simulink model "tracker"  (R2020a)
settings: Solver=VariableStepAuto  StartTime=0.0  StopTime=simulation_time  RelTol=1e-3
values from neighbouring files (symbols this model uses):
  costas_pll_arctan_nstage = 8    [tracker_hw_init.m]
  costas_pll_arctan_point = 16    [tracker_hw_init.m]
  costas_pll_arctan_width = 32    [tracker_hw_init.m]
  DDS_ch_pinc = fc.*(2^(DDS_phase_width)/fs)    [tracker_hw_init.m]
  fs = 120e6    (= 120000000)    [tracker_hw_init.m]
  normalized_EML_power_cordic_nstage = 11    [tracker_hw_init.m]
  normalized_EML_power_cordic_point = 32    [tracker_hw_init.m]
  normalized_EML_power_cordic_width = 32    [tracker_hw_init.m]
  ts = 1/fs    (= 8.33333333333e-09)    [tracker_hw_init.m]
undefined symbols (not defined in the file or in its folder): cacode, i
libraries: xbsIndex_r4 x1873
(part 2 of 14)

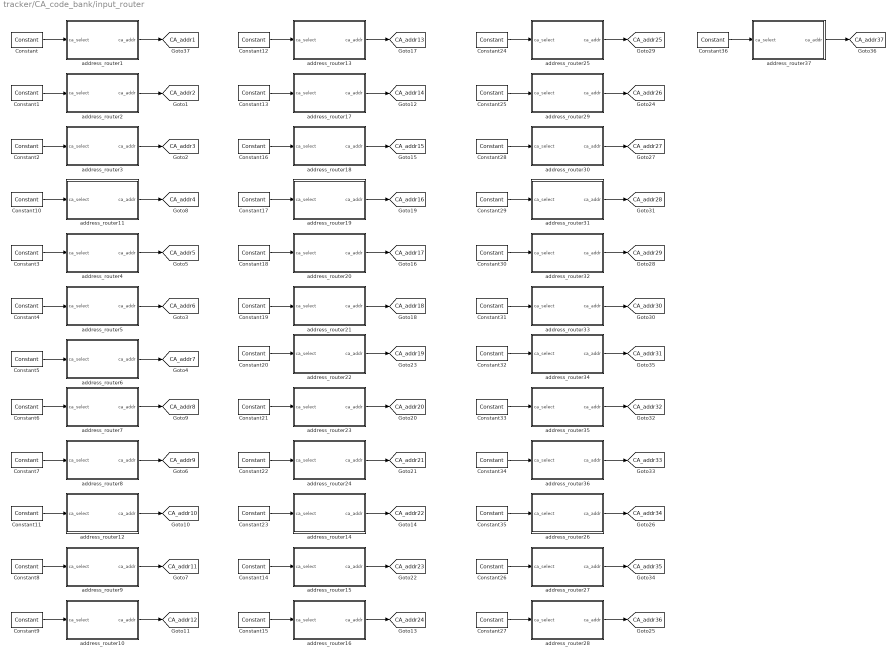
== system tracker/CA_code_bank/input_router ==
  Constant : xbsIndex_r4/Constant  const=0  gui_display_data_type=Fixed-point  arith_type=Unsigned  n_bits=6  bin_pt=0  preci_type=Single  exp_width=8  frac_width=24  explicit_period=off  period=1  equ=P=C  opselect=C  inp2=PCIN>>17  opr=+  inp1=P  carry=CIN  dbl_ovrd=off  block_type=constant
  Constant1 : xbsIndex_r4/Constant  const=1.0  gui_display_data_type=Fixed-point  arith_type=Unsigned  n_bits=6  bin_pt=0  preci_type=Single  exp_width=8  frac_width=24  explicit_period=off  period=1  equ=P=C  opselect=C  inp2=PCIN>>17  opr=+  inp1=P  carry=CIN  dbl_ovrd=off  block_type=constant
  Constant10 : xbsIndex_r4/Constant  const=3  gui_display_data_type=Fixed-point  arith_type=Unsigned  n_bits=6  bin_pt=0  preci_type=Single  exp_width=8  frac_width=24  explicit_period=off  period=1  equ=P=C  opselect=C  inp2=PCIN>>17  opr=+  inp1=P  carry=CIN  dbl_ovrd=off  block_type=constant
  Constant11 : xbsIndex_r4/Constant  const=9  gui_display_data_type=Fixed-point  arith_type=Unsigned  n_bits=6  bin_pt=0  preci_type=Single  exp_width=8  frac_width=24  explicit_period=off  period=1  equ=P=C  opselect=C  inp2=PCIN>>17  opr=+  inp1=P  carry=CIN  dbl_ovrd=off  block_type=constant
  Constant12 : xbsIndex_r4/Constant  const=12  gui_display_data_type=Fixed-point  arith_type=Unsigned  n_bits=6  bin_pt=0  preci_type=Single  exp_width=8  frac_width=24  explicit_period=off  period=1  equ=P=C  opselect=C  inp2=PCIN>>17  opr=+  inp1=P  carry=CIN  dbl_ovrd=off  block_type=constant
  Constant13 : xbsIndex_r4/Constant  const=13  gui_display_data_type=Fixed-point  arith_type=Unsigned  n_bits=6  bin_pt=0  preci_type=Single  exp_width=8  frac_width=24  explicit_period=off  period=1  equ=P=C  opselect=C  inp2=PCIN>>17  opr=+  inp1=P  carry=CIN  dbl_ovrd=off  block_type=constant
  Constant14 : xbsIndex_r4/Constant  const=22  gui_display_data_type=Fixed-point  arith_type=Unsigned  n_bits=6  bin_pt=0  preci_type=Single  exp_width=8  frac_width=24  explicit_period=off  period=1  equ=P=C  opselect=C  inp2=PCIN>>17  opr=+  inp1=P  carry=CIN  dbl_ovrd=off  block_type=constant
  Constant15 : xbsIndex_r4/Constant  const=23  gui_display_data_type=Fixed-point  arith_type=Unsigned  n_bits=6  bin_pt=0  preci_type=Single  exp_width=8  frac_width=24  explicit_period=off  period=1  equ=P=C  opselect=C  inp2=PCIN>>17  opr=+  inp1=P  carry=CIN  dbl_ovrd=off  block_type=constant
  Constant16 : xbsIndex_r4/Constant  const=14  gui_display_data_type=Fixed-point  arith_type=Unsigned  n_bits=6  bin_pt=0  preci_type=Single  exp_width=8  frac_width=24  explicit_period=off  period=1  equ=P=C  opselect=C  inp2=PCIN>>17  opr=+  inp1=P  carry=CIN  dbl_ovrd=off  block_type=constant
  Constant17 : xbsIndex_r4/Constant  const=15  gui_display_data_type=Fixed-point  arith_type=Unsigned  n_bits=6  bin_pt=0  preci_type=Single  exp_width=8  frac_width=24  explicit_period=off  period=1  equ=P=C  opselect=C  inp2=PCIN>>17  opr=+  inp1=P  carry=CIN  dbl_ovrd=off  block_type=constant
  Constant18 : xbsIndex_r4/Constant  const=16  gui_display_data_type=Fixed-point  arith_type=Unsigned  n_bits=6  bin_pt=0  preci_type=Single  exp_width=8  frac_width=24  explicit_period=off  period=1  equ=P=C  opselect=C  inp2=PCIN>>17  opr=+  inp1=P  carry=CIN  dbl_ovrd=off  block_type=constant
  Constant19 : xbsIndex_r4/Constant  const=17  gui_display_data_type=Fixed-point  arith_type=Unsigned  n_bits=6  bin_pt=0  preci_type=Single  exp_width=8  frac_width=24  explicit_period=off  period=1  equ=P=C  opselect=C  inp2=PCIN>>17  opr=+  inp1=P  carry=CIN  dbl_ovrd=off  block_type=constant
  Constant2 : xbsIndex_r4/Constant  const=2  gui_display_data_type=Fixed-point  arith_type=Unsigned  n_bits=6  bin_pt=0  preci_type=Single  exp_width=8  frac_width=24  explicit_period=off  period=1  equ=P=C  opselect=C  inp2=PCIN>>17  opr=+  inp1=P  carry=CIN  dbl_ovrd=off  block_type=constant
  Constant20 : xbsIndex_r4/Constant  const=18  gui_display_data_type=Fixed-point  arith_type=Unsigned  n_bits=6  bin_pt=0  preci_type=Single  exp_width=8  frac_width=24  explicit_period=off  period=1  equ=P=C  opselect=C  inp2=PCIN>>17  opr=+  inp1=P  carry=CIN  dbl_ovrd=off  block_type=constant
  Constant21 : xbsIndex_r4/Constant  const=19  gui_display_data_type=Fixed-point  arith_type=Unsigned  n_bits=6  bin_pt=0  preci_type=Single  exp_width=8  frac_width=24  explicit_period=off  period=1  equ=P=C  opselect=C  inp2=PCIN>>17  opr=+  inp1=P  carry=CIN  dbl_ovrd=off  block_type=constant
  Constant22 : xbsIndex_r4/Constant  const=20  gui_display_data_type=Fixed-point  arith_type=Unsigned  n_bits=6  bin_pt=0  preci_type=Single  exp_width=8  frac_width=24  explicit_period=off  period=1  equ=P=C  opselect=C  inp2=PCIN>>17  opr=+  inp1=P  carry=CIN  dbl_ovrd=off  block_type=constant
  Constant23 : xbsIndex_r4/Constant  const=21  gui_display_data_type=Fixed-point  arith_type=Unsigned  n_bits=6  bin_pt=0  preci_type=Single  exp_width=8  frac_width=24  explicit_period=off  period=1  equ=P=C  opselect=C  inp2=PCIN>>17  opr=+  inp1=P  carry=CIN  dbl_ovrd=off  block_type=constant
  Constant24 : xbsIndex_r4/Constant  const=24  gui_display_data_type=Fixed-point  arith_type=Unsigned  n_bits=6  bin_pt=0  preci_type=Single  exp_width=8  frac_width=24  explicit_period=off  period=1  equ=P=C  opselect=C  inp2=PCIN>>17  opr=+  inp1=P  carry=CIN  dbl_ovrd=off  block_type=constant
  Constant25 : xbsIndex_r4/Constant  const=25  gui_display_data_type=Fixed-point  arith_type=Unsigned  n_bits=6  bin_pt=0  preci_type=Single  exp_width=8  frac_width=24  explicit_period=off  period=1  equ=P=C  opselect=C  inp2=PCIN>>17  opr=+  inp1=P  carry=CIN  dbl_ovrd=off  block_type=constant
  Constant26 : xbsIndex_r4/Constant  const=34  gui_display_data_type=Fixed-point  arith_type=Unsigned  n_bits=6  bin_pt=0  preci_type=Single  exp_width=8  frac_width=24  explicit_period=off  period=1  equ=P=C  opselect=C  inp2=PCIN>>17  opr=+  inp1=P  carry=CIN  dbl_ovrd=off  block_type=constant
  Constant27 : xbsIndex_r4/Constant  const=35  gui_display_data_type=Fixed-point  arith_type=Unsigned  n_bits=6  bin_pt=0  preci_type=Single  exp_width=8  frac_width=24  explicit_period=off  period=1  equ=P=C  opselect=C  inp2=PCIN>>17  opr=+  inp1=P  carry=CIN  dbl_ovrd=off  block_type=constant
  Constant28 : xbsIndex_r4/Constant  const=26  gui_display_data_type=Fixed-point  arith_type=Unsigned  n_bits=6  bin_pt=0  preci_type=Single  exp_width=8  frac_width=24  explicit_period=off  period=1  equ=P=C  opselect=C  inp2=PCIN>>17  opr=+  inp1=P  carry=CIN  dbl_ovrd=off  block_type=constant
  Constant29 : xbsIndex_r4/Constant  const=27  gui_display_data_type=Fixed-point  arith_type=Unsigned  n_bits=6  bin_pt=0  preci_type=Single  exp_width=8  frac_width=24  explicit_period=off  period=1  equ=P=C  opselect=C  inp2=PCIN>>17  opr=+  inp1=P  carry=CIN  dbl_ovrd=off  block_type=constant
  Constant3 : xbsIndex_r4/Constant  const=4  gui_display_data_type=Fixed-point  arith_type=Unsigned  n_bits=6  bin_pt=0  preci_type=Single  exp_width=8  frac_width=24  explicit_period=off  period=1  equ=P=C  opselect=C  inp2=PCIN>>17  opr=+  inp1=P  carry=CIN  dbl_ovrd=off  block_type=constant
  Constant30 : xbsIndex_r4/Constant  const=28  gui_display_data_type=Fixed-point  arith_type=Unsigned  n_bits=6  bin_pt=0  preci_type=Single  exp_width=8  frac_width=24  explicit_period=off  period=1  equ=P=C  opselect=C  inp2=PCIN>>17  opr=+  inp1=P  carry=CIN  dbl_ovrd=off  block_type=constant
  Constant31 : xbsIndex_r4/Constant  const=29  gui_display_data_type=Fixed-point  arith_type=Unsigned  n_bits=6  bin_pt=0  preci_type=Single  exp_width=8  frac_width=24  explicit_period=off  period=1  equ=P=C  opselect=C  inp2=PCIN>>17  opr=+  inp1=P  carry=CIN  dbl_ovrd=off  block_type=constant
  Constant32 : xbsIndex_r4/Constant  const=30  gui_display_data_type=Fixed-point  arith_type=Unsigned  n_bits=6  bin_pt=0  preci_type=Single  exp_width=8  frac_width=24  explicit_period=off  period=1  equ=P=C  opselect=C  inp2=PCIN>>17  opr=+  inp1=P  carry=CIN  dbl_ovrd=off  block_type=constant
  Constant33 : xbsIndex_r4/Constant  const=31  gui_display_data_type=Fixed-point  arith_type=Unsigned  n_bits=6  bin_pt=0  preci_type=Single  exp_width=8  frac_width=24  explicit_period=off  period=1  equ=P=C  opselect=C  inp2=PCIN>>17  opr=+  inp1=P  carry=CIN  dbl_ovrd=off  block_type=constant
  Constant34 : xbsIndex_r4/Constant  const=32  gui_display_data_type=Fixed-point  arith_type=Unsigned  n_bits=6  bin_pt=0  preci_type=Single  exp_width=8  frac_width=24  explicit_period=off  period=1  equ=P=C  opselect=C  inp2=PCIN>>17  opr=+  inp1=P  carry=CIN  dbl_ovrd=off  block_type=constant
  Constant35 : xbsIndex_r4/Constant  const=33  gui_display_data_type=Fixed-point  arith_type=Unsigned  n_bits=6  bin_pt=0  preci_type=Single  exp_width=8  frac_width=24  explicit_period=off  period=1  equ=P=C  opselect=C  inp2=PCIN>>17  opr=+  inp1=P  carry=CIN  dbl_ovrd=off  block_type=constant
  Constant36 : xbsIndex_r4/Constant  const=36  gui_display_data_type=Fixed-point  arith_type=Unsigned  n_bits=6  bin_pt=0  preci_type=Single  exp_width=8  frac_width=24  explicit_period=off  period=1  equ=P=C  opselect=C  inp2=PCIN>>17  opr=+  inp1=P  carry=CIN  dbl_ovrd=off  block_type=constant
  Constant4 : xbsIndex_r4/Constant  const=5  gui_display_data_type=Fixed-point  arith_type=Unsigned  n_bits=6  bin_pt=0  preci_type=Single  exp_width=8  frac_width=24  explicit_period=off  period=1  equ=P=C  opselect=C  inp2=PCIN>>17  opr=+  inp1=P  carry=CIN  dbl_ovrd=off  block_type=constant
  Constant5 : xbsIndex_r4/Constant  const=6  gui_display_data_type=Fixed-point  arith_type=Unsigned  n_bits=6  bin_pt=0  preci_type=Single  exp_width=8  frac_width=24  explicit_period=off  period=1  equ=P=C  opselect=C  inp2=PCIN>>17  opr=+  inp1=P  carry=CIN  dbl_ovrd=off  block_type=constant
  Constant6 : xbsIndex_r4/Constant  const=7  gui_display_data_type=Fixed-point  arith_type=Unsigned  n_bits=6  bin_pt=0  preci_type=Single  exp_width=8  frac_width=24  explicit_period=off  period=1  equ=P=C  opselect=C  inp2=PCIN>>17  opr=+  inp1=P  carry=CIN  dbl_ovrd=off  block_type=constant
  Constant7 : xbsIndex_r4/Constant  const=8  gui_display_data_type=Fixed-point  arith_type=Unsigned  n_bits=6  bin_pt=0  preci_type=Single  exp_width=8  frac_width=24  explicit_period=off  period=1  equ=P=C  opselect=C  inp2=PCIN>>17  opr=+  inp1=P  carry=CIN  dbl_ovrd=off  block_type=constant
  Constant8 : xbsIndex_r4/Constant  const=10  gui_display_data_type=Fixed-point  arith_type=Unsigned  n_bits=6  bin_pt=0  preci_type=Single  exp_width=8  frac_width=24  explicit_period=off  period=1  equ=P=C  opselect=C  inp2=PCIN>>17  opr=+  inp1=P  carry=CIN  dbl_ovrd=off  block_type=constant
  Constant9 : xbsIndex_r4/Constant  const=11  gui_display_data_type=Fixed-point  arith_type=Unsigned  n_bits=6  bin_pt=0  preci_type=Single  exp_width=8  frac_width=24  explicit_period=off  period=1  equ=P=C  opselect=C  inp2=PCIN>>17  opr=+  inp1=P  carry=CIN  dbl_ovrd=off  block_type=constant
  address_router1 : Subsystem
  address_router10 : Subsystem
  address_router11 : Subsystem
  address_router12 : Subsystem
  address_router13 : Subsystem
  address_router14 : Subsystem
  address_router15 : Subsystem
  address_router16 : Subsystem
  address_router17 : Subsystem
  address_router18 : Subsystem
  address_router19 : Subsystem
  address_router2 : Subsystem
  address_router20 : Subsystem
  address_router21 : Subsystem
  address_router22 : Subsystem
  address_router23 : Subsystem
  address_router24 : Subsystem
  address_router25 : Subsystem
  address_router26 : Subsystem
  address_router27 : Subsystem
  address_router28 : Subsystem
  address_router29 : Subsystem
  address_router3 : Subsystem
  address_router30 : Subsystem
  address_router31 : Subsystem
  address_router32 : Subsystem
  address_router33 : Subsystem
  address_router34 : Subsystem
  address_router35 : Subsystem
  address_router36 : Subsystem
  address_router37 : Subsystem
  address_router4 : Subsystem
  address_router5 : Subsystem
  address_router6 : Subsystem
  address_router7 : Subsystem
  address_router8 : Subsystem
  address_router9 : Subsystem
  tag scope: CA_addr10=global, CA_addr11=global, CA_addr12=global, CA_addr13=global, CA_addr14=global, CA_addr15=global, CA_addr16=global, CA_addr17=global, CA_addr18=global, CA_addr19=global, CA_addr1=global, CA_addr20=global, CA_addr21=global, CA_addr22=global, CA_addr23=global, CA_addr24=global, CA_addr25=global, CA_addr26=global, CA_addr27=global, CA_addr28=global, CA_addr29=global, CA_addr2=global, CA_addr30=global, CA_addr31=global, CA_addr32=global, CA_addr33=global, CA_addr34=global, CA_addr35=global, CA_addr36=global, CA_addr37=global, CA_addr3=global, CA_addr4=global, CA_addr5=global, CA_addr6=global, CA_addr7=global, CA_addr8=global, CA_addr9=global
  wires:
  address_router1/1(ca_addr) -> [CA_addr1]
  Constant/1 -> address_router1/1(ca_select)
  address_router2/1(ca_addr) -> [CA_addr2]
  Constant1/1 -> address_router2/1(ca_select)
  Constant2/1 -> address_router3/1(ca_select)
  address_router3/1(ca_addr) -> [CA_addr3]
  address_router6/1(ca_addr) -> [CA_addr7]
  Constant5/1 -> address_router6/1(ca_select)
  Constant4/1 -> address_router5/1(ca_select)
  address_router5/1(ca_addr) -> [CA_addr6]
  Constant3/1 -> address_router4/1(ca_select)
  address_router4/1(ca_addr) -> [CA_addr5]
  address_router10/1(ca_addr) -> [CA_addr12]
  Constant9/1 -> address_router10/1(ca_select)
  address_router11/1(ca_addr) -> [CA_addr4]
  Constant10/1 -> address_router11/1(ca_select)
  Constant11/1 -> address_router12/1(ca_select)
  address_router12/1(ca_addr) -> [CA_addr10]
  address_router9/1(ca_addr) -> [CA_addr11]
  Constant8/1 -> address_router9/1(ca_select)
  Constant7/1 -> address_router8/1(ca_select)
  address_router8/1(ca_addr) -> [CA_addr9]
  Constant6/1 -> address_router7/1(ca_select)
  address_router7/1(ca_addr) -> [CA_addr8]
  address_router22/1(ca_addr) -> [CA_addr19]
  Constant20/1 -> address_router22/1(ca_select)
  address_router23/1(ca_addr) -> [CA_addr20]
  Constant21/1 -> address_router23/1(ca_select)
  Constant22/1 -> address_router24/1(ca_select)
  address_router24/1(ca_addr) -> [CA_addr21]
  address_router16/1(ca_addr) -> [CA_addr24]
  Constant15/1 -> address_router16/1(ca_select)
  Constant14/1 -> address_router15/1(ca_select)
  address_router15/1(ca_addr) -> [CA_addr23]
  Constant23/1 -> address_router14/1(ca_select)
  address_router14/1(ca_addr) -> [CA_addr22]
  address_router19/1(ca_addr) -> [CA_addr16]
  Constant17/1 -> address_router19/1(ca_select)
  address_router20/1(ca_addr) -> [CA_addr17]
  Constant18/1 -> address_router20/1(ca_select)
  Constant19/1 -> address_router21/1(ca_select)
  address_router21/1(ca_addr) -> [CA_addr18]
  address_router18/1(ca_addr) -> [CA_addr15]
  Constant16/1 -> address_router18/1(ca_select)
  Constant13/1 -> address_router17/1(ca_select)
  address_router17/1(ca_addr) -> [CA_addr14]
  Constant12/1 -> address_router13/1(ca_select)
  address_router13/1(ca_addr) -> [CA_addr13]
  address_router25/1(ca_addr) -> [CA_addr25]
  Constant24/1 -> address_router25/1(ca_select)
  address_router29/1(ca_addr) -> [CA_addr26]
  Constant25/1 -> address_router29/1(ca_select)
  Constant28/1 -> address_router30/1(ca_select)
  address_router30/1(ca_addr) -> [CA_addr27]
  address_router33/1(ca_addr) -> [CA_addr30]
  Constant31/1 -> address_router33/1(ca_select)
  Constant30/1 -> address_router32/1(ca_select)
  address_router32/1(ca_addr) -> [CA_addr29]
  Constant29/1 -> address_router31/1(ca_select)
  address_router31/1(ca_addr) -> [CA_addr28]
  address_router26/1(ca_addr) -> [CA_addr34]
  Constant35/1 -> address_router26/1(ca_select)
  address_router27/1(ca_addr) -> [CA_addr35]
  Constant26/1 -> address_router27/1(ca_select)
  Constant27/1 -> address_router28/1(ca_select)
  address_router28/1(ca_addr) -> [CA_addr36]
  address_router36/1(ca_addr) -> [CA_addr33]
  Constant34/1 -> address_router36/1(ca_select)
  Constant33/1 -> address_router35/1(ca_select)
  address_router35/1(ca_addr) -> [CA_addr32]
  Constant32/1 -> address_router34/1(ca_select)
  address_router34/1(ca_addr) -> [CA_addr31]
  Constant36/1 -> address_router37/1(ca_select)
  address_router37/1(ca_addr) -> [CA_addr37]

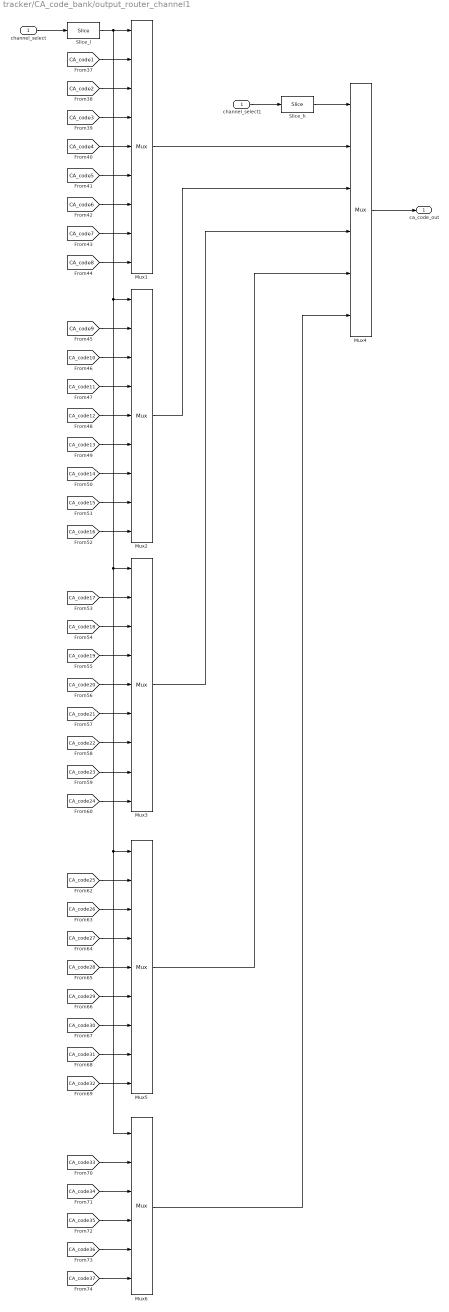
== system tracker/CA_code_bank/output_router_channel1 ==
  channel_select : Inport
  Mux{1..3,5} (4 alike) : xbsIndex_r4/Mux  inputs=8  en=off  latency=1  precision=Full  arith_type=Unsigned  n_bits=16  bin_pt=14  quantization=Truncate  overflow=Wrap  dbl_ovrd=off  block_type=mux
  Mux4 : xbsIndex_r4/Mux  inputs=5  en=off  latency=1  precision=Full  arith_type=Unsigned  n_bits=16  bin_pt=14  quantization=Truncate  overflow=Wrap  dbl_ovrd=off  block_type=mux
  Mux6 : xbsIndex_r4/Mux  inputs=5  en=off  latency=1  precision=Full  arith_type=Unsigned  n_bits=16  bin_pt=14  quantization=Truncate  overflow=Wrap  dbl_ovrd=off  block_type=mux
  Slice_h : xbsIndex_r4/Slice  nbits=3  boolean_output=off  mode=Lower Bit Location + Width  bit1=0  base1=MSB of Input  bit0=3  base0=LSB of Input  dbl_ovrd=off  block_type=slice
  Slice_l : xbsIndex_r4/Slice  nbits=3  boolean_output=off  mode=Lower Bit Location + Width  bit1=0  base1=MSB of Input  bit0=0  base0=LSB of Input  dbl_ovrd=off  block_type=slice
  channel_select1 : InportShadow
  ca_code_out : Outport
  wires:
  [CA_code10] -> Mux2/3
  [CA_code1] -> Mux1/2
  [CA_code18] -> Mux3/3
  [CA_code11] -> Mux2/4
  Mux6/1 -> Mux4/6
  [CA_code36] -> Mux6/5
  [CA_code16] -> Mux2/9
  [CA_code25] -> Mux5/2
  [CA_code3] -> Mux1/4
  [CA_code28] -> Mux5/5
  [CA_code33] -> Mux6/2
  [CA_code13] -> Mux2/6
  Mux2/1 -> Mux4/3
  [CA_code27] -> Mux5/4
  [CA_code35] -> Mux6/4
  [CA_code5] -> Mux1/6
  [CA_code4] -> Mux1/5
  [CA_code6] -> Mux1/7
  [CA_code8] -> Mux1/9
  [CA_code20] -> Mux3/5
  Mux4/1 -> ca_code_out/1
  [CA_code9] -> Mux2/2
  Mux3/1 -> Mux4/4
  [CA_code34] -> Mux6/3
  [CA_code22] -> Mux3/7
  [CA_code30] -> Mux5/7
  [CA_code37] -> Mux6/6
  [CA_code23] -> Mux3/8
  [CA_code19] -> Mux3/4
  [CA_code2] -> Mux1/3
  [CA_code24] -> Mux3/9
  [CA_code31] -> Mux5/8
  [CA_code26] -> Mux5/3
  Mux1/1 -> Mux4/2
  [CA_code21] -> Mux3/6
  Mux5/1 -> Mux4/5
  [CA_code29] -> Mux5/6
  [CA_code14] -> Mux2/7
  [CA_code12] -> Mux2/5
  [CA_code7] -> Mux1/8
  [CA_code15] -> Mux2/8
  [CA_code32] -> Mux5/9
  [CA_code17] -> Mux3/2
  Slice_l/1 -> Mux2/1, Mux3/1, Mux5/1, Mux6/1, Mux1/1
  channel_select/1 -> Slice_l/1
  channel_select1/1 -> Slice_h/1
  Slice_h/1 -> Mux4/1

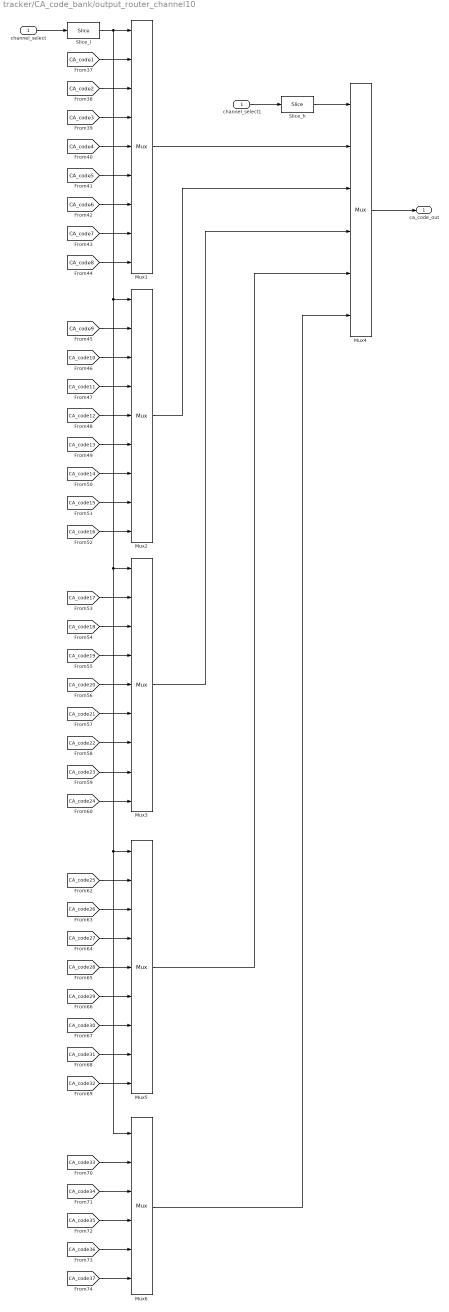
== system tracker/CA_code_bank/output_router_channel10 ==
  channel_select : Inport
  Mux{1..3,5} (4 alike) : xbsIndex_r4/Mux  inputs=8  en=off  latency=1  precision=Full  arith_type=Unsigned  n_bits=16  bin_pt=14  quantization=Truncate  overflow=Wrap  dbl_ovrd=off  block_type=mux
  Mux4 : xbsIndex_r4/Mux  inputs=5  en=off  latency=1  precision=Full  arith_type=Unsigned  n_bits=16  bin_pt=14  quantization=Truncate  overflow=Wrap  dbl_ovrd=off  block_type=mux
  Mux6 : xbsIndex_r4/Mux  inputs=5  en=off  latency=1  precision=Full  arith_type=Unsigned  n_bits=16  bin_pt=14  quantization=Truncate  overflow=Wrap  dbl_ovrd=off  block_type=mux
  Slice_h : xbsIndex_r4/Slice  nbits=3  boolean_output=off  mode=Lower Bit Location + Width  bit1=0  base1=MSB of Input  bit0=3  base0=LSB of Input  dbl_ovrd=off  block_type=slice
  Slice_l : xbsIndex_r4/Slice  nbits=3  boolean_output=off  mode=Lower Bit Location + Width  bit1=0  base1=MSB of Input  bit0=0  base0=LSB of Input  dbl_ovrd=off  block_type=slice
  channel_select1 : InportShadow
  ca_code_out : Outport
  wires:
  [CA_code10] -> Mux2/3
  [CA_code1] -> Mux1/2
  [CA_code18] -> Mux3/3
  [CA_code11] -> Mux2/4
  Mux6/1 -> Mux4/6
  [CA_code36] -> Mux6/5
  [CA_code16] -> Mux2/9
  [CA_code25] -> Mux5/2
  [CA_code3] -> Mux1/4
  [CA_code28] -> Mux5/5
  [CA_code33] -> Mux6/2
  [CA_code13] -> Mux2/6
  Mux2/1 -> Mux4/3
  [CA_code27] -> Mux5/4
  [CA_code35] -> Mux6/4
  [CA_code5] -> Mux1/6
  [CA_code4] -> Mux1/5
  [CA_code6] -> Mux1/7
  [CA_code8] -> Mux1/9
  [CA_code20] -> Mux3/5
  Mux4/1 -> ca_code_out/1
  [CA_code9] -> Mux2/2
  Mux3/1 -> Mux4/4
  [CA_code34] -> Mux6/3
  [CA_code22] -> Mux3/7
  [CA_code30] -> Mux5/7
  [CA_code37] -> Mux6/6
  [CA_code23] -> Mux3/8
  [CA_code19] -> Mux3/4
  [CA_code2] -> Mux1/3
  [CA_code24] -> Mux3/9
  [CA_code31] -> Mux5/8
  [CA_code26] -> Mux5/3
  Mux1/1 -> Mux4/2
  [CA_code21] -> Mux3/6
  Mux5/1 -> Mux4/5
  [CA_code29] -> Mux5/6
  [CA_code14] -> Mux2/7
  [CA_code12] -> Mux2/5
  [CA_code7] -> Mux1/8
  [CA_code15] -> Mux2/8
  [CA_code32] -> Mux5/9
  [CA_code17] -> Mux3/2
  Slice_l/1 -> Mux2/1, Mux3/1, Mux5/1, Mux6/1, Mux1/1
  channel_select/1 -> Slice_l/1
  channel_select1/1 -> Slice_h/1
  Slice_h/1 -> Mux4/1

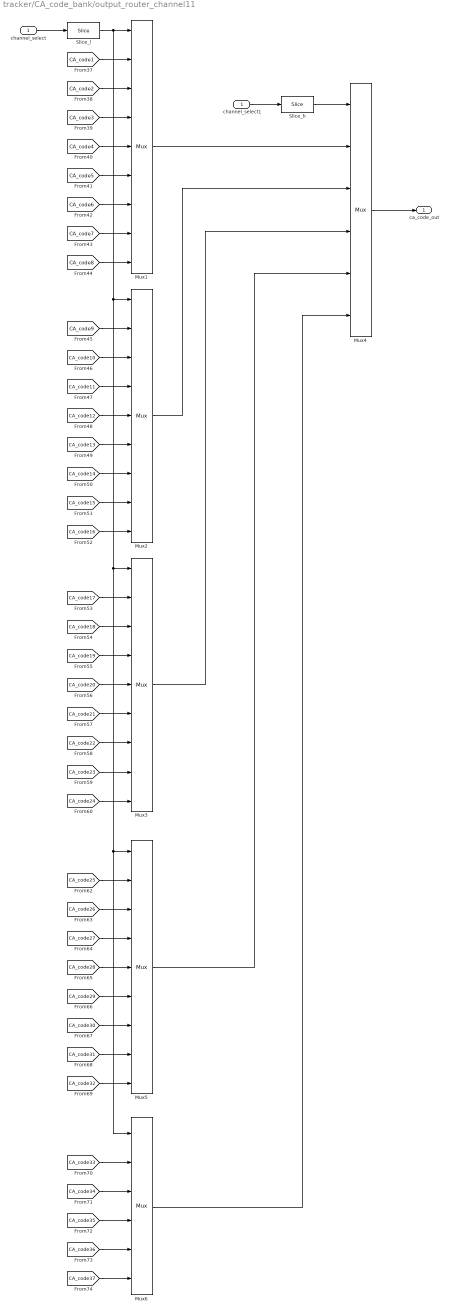
== system tracker/CA_code_bank/output_router_channel11 ==
  channel_select : Inport
  Mux{1..3,5} (4 alike) : xbsIndex_r4/Mux  inputs=8  en=off  latency=1  precision=Full  arith_type=Unsigned  n_bits=16  bin_pt=14  quantization=Truncate  overflow=Wrap  dbl_ovrd=off  block_type=mux
  Mux4 : xbsIndex_r4/Mux  inputs=5  en=off  latency=1  precision=Full  arith_type=Unsigned  n_bits=16  bin_pt=14  quantization=Truncate  overflow=Wrap  dbl_ovrd=off  block_type=mux
  Mux6 : xbsIndex_r4/Mux  inputs=5  en=off  latency=1  precision=Full  arith_type=Unsigned  n_bits=16  bin_pt=14  quantization=Truncate  overflow=Wrap  dbl_ovrd=off  block_type=mux
  Slice_h : xbsIndex_r4/Slice  nbits=3  boolean_output=off  mode=Lower Bit Location + Width  bit1=0  base1=MSB of Input  bit0=3  base0=LSB of Input  dbl_ovrd=off  block_type=slice
  Slice_l : xbsIndex_r4/Slice  nbits=3  boolean_output=off  mode=Lower Bit Location + Width  bit1=0  base1=MSB of Input  bit0=0  base0=LSB of Input  dbl_ovrd=off  block_type=slice
  channel_select1 : InportShadow
  ca_code_out : Outport
  wires:
  Slice_h/1 -> Mux4/1
  channel_select1/1 -> Slice_h/1
  channel_select/1 -> Slice_l/1
  Slice_l/1 -> Mux1/1, Mux6/1, Mux5/1, Mux3/1, Mux2/1
  [CA_code17] -> Mux3/2
  [CA_code32] -> Mux5/9
  [CA_code15] -> Mux2/8
  [CA_code7] -> Mux1/8
  [CA_code12] -> Mux2/5
  [CA_code14] -> Mux2/7
  [CA_code29] -> Mux5/6
  Mux5/1 -> Mux4/5
  [CA_code21] -> Mux3/6
  Mux1/1 -> Mux4/2
  [CA_code26] -> Mux5/3
  [CA_code31] -> Mux5/8
  [CA_code24] -> Mux3/9
  [CA_code2] -> Mux1/3
  [CA_code19] -> Mux3/4
  [CA_code23] -> Mux3/8
  [CA_code37] -> Mux6/6
  [CA_code30] -> Mux5/7
  [CA_code22] -> Mux3/7
  [CA_code34] -> Mux6/3
  Mux3/1 -> Mux4/4
  [CA_code9] -> Mux2/2
  Mux4/1 -> ca_code_out/1
  [CA_code20] -> Mux3/5
  [CA_code8] -> Mux1/9
  [CA_code6] -> Mux1/7
  [CA_code4] -> Mux1/5
  [CA_code5] -> Mux1/6
  [CA_code35] -> Mux6/4
  [CA_code27] -> Mux5/4
  Mux2/1 -> Mux4/3
  [CA_code13] -> Mux2/6
  [CA_code33] -> Mux6/2
  [CA_code28] -> Mux5/5
  [CA_code3] -> Mux1/4
  [CA_code25] -> Mux5/2
  [CA_code16] -> Mux2/9
  [CA_code36] -> Mux6/5
  Mux6/1 -> Mux4/6
  [CA_code11] -> Mux2/4
  [CA_code18] -> Mux3/3
  [CA_code1] -> Mux1/2
  [CA_code10] -> Mux2/3

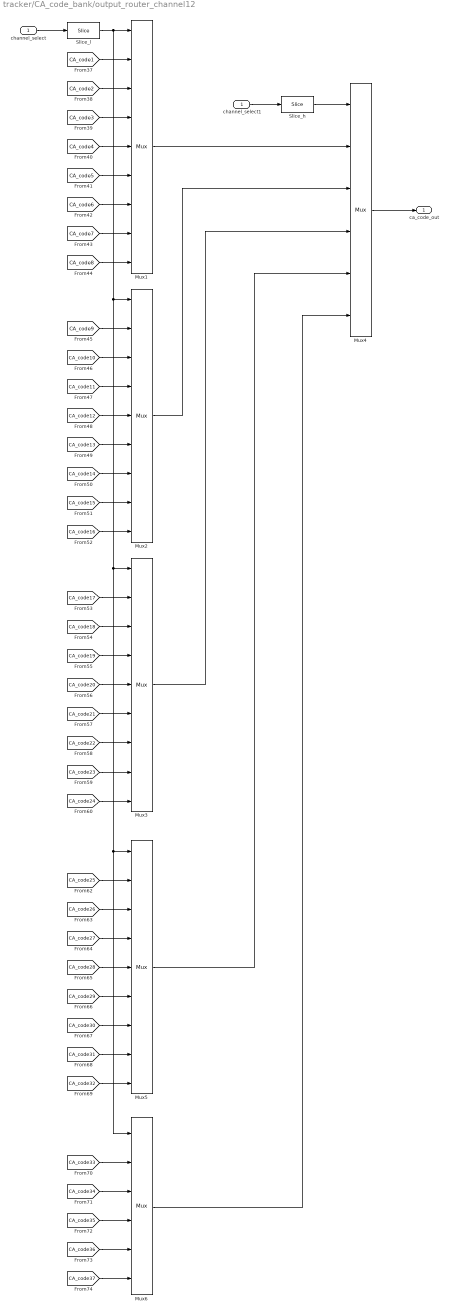
== system tracker/CA_code_bank/output_router_channel12 ==
  channel_select : Inport
  Mux{1..3,5} (4 alike) : xbsIndex_r4/Mux  inputs=8  en=off  latency=1  precision=Full  arith_type=Unsigned  n_bits=16  bin_pt=14  quantization=Truncate  overflow=Wrap  dbl_ovrd=off  block_type=mux
  Mux4 : xbsIndex_r4/Mux  inputs=5  en=off  latency=1  precision=Full  arith_type=Unsigned  n_bits=16  bin_pt=14  quantization=Truncate  overflow=Wrap  dbl_ovrd=off  block_type=mux
  Mux6 : xbsIndex_r4/Mux  inputs=5  en=off  latency=1  precision=Full  arith_type=Unsigned  n_bits=16  bin_pt=14  quantization=Truncate  overflow=Wrap  dbl_ovrd=off  block_type=mux
  Slice_h : xbsIndex_r4/Slice  nbits=3  boolean_output=off  mode=Lower Bit Location + Width  bit1=0  base1=MSB of Input  bit0=3  base0=LSB of Input  dbl_ovrd=off  block_type=slice
  Slice_l : xbsIndex_r4/Slice  nbits=3  boolean_output=off  mode=Lower Bit Location + Width  bit1=0  base1=MSB of Input  bit0=0  base0=LSB of Input  dbl_ovrd=off  block_type=slice
  channel_select1 : InportShadow
  ca_code_out : Outport
  wires:
  [CA_code10] -> Mux2/3
  [CA_code1] -> Mux1/2
  [CA_code18] -> Mux3/3
  [CA_code11] -> Mux2/4
  Mux6/1 -> Mux4/6
  [CA_code36] -> Mux6/5
  [CA_code16] -> Mux2/9
  [CA_code25] -> Mux5/2
  [CA_code3] -> Mux1/4
  [CA_code28] -> Mux5/5
  [CA_code33] -> Mux6/2
  [CA_code13] -> Mux2/6
  Mux2/1 -> Mux4/3
  [CA_code27] -> Mux5/4
  [CA_code35] -> Mux6/4
  [CA_code5] -> Mux1/6
  [CA_code4] -> Mux1/5
  [CA_code6] -> Mux1/7
  [CA_code8] -> Mux1/9
  [CA_code20] -> Mux3/5
  Mux4/1 -> ca_code_out/1
  [CA_code9] -> Mux2/2
  Mux3/1 -> Mux4/4
  [CA_code34] -> Mux6/3
  [CA_code22] -> Mux3/7
  [CA_code30] -> Mux5/7
  [CA_code37] -> Mux6/6
  [CA_code23] -> Mux3/8
  [CA_code19] -> Mux3/4
  [CA_code2] -> Mux1/3
  [CA_code24] -> Mux3/9
  [CA_code31] -> Mux5/8
  [CA_code26] -> Mux5/3
  Mux1/1 -> Mux4/2
  [CA_code21] -> Mux3/6
  Mux5/1 -> Mux4/5
  [CA_code29] -> Mux5/6
  [CA_code14] -> Mux2/7
  [CA_code12] -> Mux2/5
  [CA_code7] -> Mux1/8
  [CA_code15] -> Mux2/8
  [CA_code32] -> Mux5/9
  [CA_code17] -> Mux3/2
  Slice_l/1 -> Mux2/1, Mux3/1, Mux5/1, Mux6/1, Mux1/1
  channel_select/1 -> Slice_l/1
  channel_select1/1 -> Slice_h/1
  Slice_h/1 -> Mux4/1

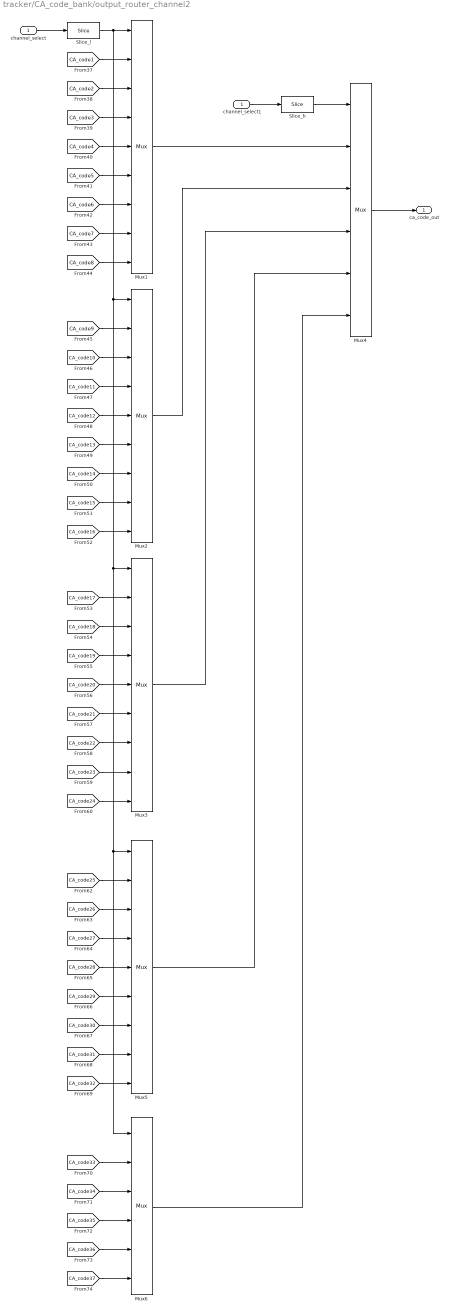
== system tracker/CA_code_bank/output_router_channel2 ==
  channel_select : Inport
  Mux{1..3,5} (4 alike) : xbsIndex_r4/Mux  inputs=8  en=off  latency=1  precision=Full  arith_type=Unsigned  n_bits=16  bin_pt=14  quantization=Truncate  overflow=Wrap  dbl_ovrd=off  block_type=mux
  Mux4 : xbsIndex_r4/Mux  inputs=5  en=off  latency=1  precision=Full  arith_type=Unsigned  n_bits=16  bin_pt=14  quantization=Truncate  overflow=Wrap  dbl_ovrd=off  block_type=mux
  Mux6 : xbsIndex_r4/Mux  inputs=5  en=off  latency=1  precision=Full  arith_type=Unsigned  n_bits=16  bin_pt=14  quantization=Truncate  overflow=Wrap  dbl_ovrd=off  block_type=mux
  Slice_h : xbsIndex_r4/Slice  nbits=3  boolean_output=off  mode=Lower Bit Location + Width  bit1=0  base1=MSB of Input  bit0=3  base0=LSB of Input  dbl_ovrd=off  block_type=slice
  Slice_l : xbsIndex_r4/Slice  nbits=3  boolean_output=off  mode=Lower Bit Location + Width  bit1=0  base1=MSB of Input  bit0=0  base0=LSB of Input  dbl_ovrd=off  block_type=slice
  channel_select1 : InportShadow
  ca_code_out : Outport
  wires:
  Slice_h/1 -> Mux4/1
  channel_select1/1 -> Slice_h/1
  channel_select/1 -> Slice_l/1
  Slice_l/1 -> Mux1/1, Mux6/1, Mux5/1, Mux3/1, Mux2/1
  [CA_code17] -> Mux3/2
  [CA_code32] -> Mux5/9
  [CA_code15] -> Mux2/8
  [CA_code7] -> Mux1/8
  [CA_code12] -> Mux2/5
  [CA_code14] -> Mux2/7
  [CA_code29] -> Mux5/6
  Mux5/1 -> Mux4/5
  [CA_code21] -> Mux3/6
  Mux1/1 -> Mux4/2
  [CA_code26] -> Mux5/3
  [CA_code31] -> Mux5/8
  [CA_code24] -> Mux3/9
  [CA_code2] -> Mux1/3
  [CA_code19] -> Mux3/4
  [CA_code23] -> Mux3/8
  [CA_code37] -> Mux6/6
  [CA_code30] -> Mux5/7
  [CA_code22] -> Mux3/7
  [CA_code34] -> Mux6/3
  Mux3/1 -> Mux4/4
  [CA_code9] -> Mux2/2
  Mux4/1 -> ca_code_out/1
  [CA_code20] -> Mux3/5
  [CA_code8] -> Mux1/9
  [CA_code6] -> Mux1/7
  [CA_code4] -> Mux1/5
  [CA_code5] -> Mux1/6
  [CA_code35] -> Mux6/4
  [CA_code27] -> Mux5/4
  Mux2/1 -> Mux4/3
  [CA_code13] -> Mux2/6
  [CA_code33] -> Mux6/2
  [CA_code28] -> Mux5/5
  [CA_code3] -> Mux1/4
  [CA_code25] -> Mux5/2
  [CA_code16] -> Mux2/9
  [CA_code36] -> Mux6/5
  Mux6/1 -> Mux4/6
  [CA_code11] -> Mux2/4
  [CA_code18] -> Mux3/3
  [CA_code1] -> Mux1/2
  [CA_code10] -> Mux2/3

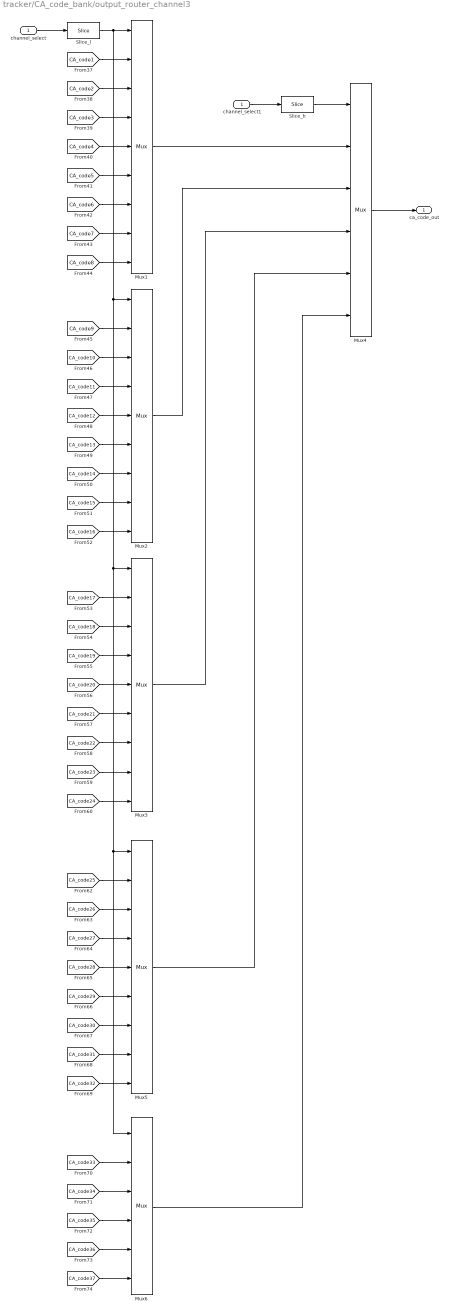
== system tracker/CA_code_bank/output_router_channel3 ==
  channel_select : Inport
  Mux{1..3,5} (4 alike) : xbsIndex_r4/Mux  inputs=8  en=off  latency=1  precision=Full  arith_type=Unsigned  n_bits=16  bin_pt=14  quantization=Truncate  overflow=Wrap  dbl_ovrd=off  block_type=mux
  Mux4 : xbsIndex_r4/Mux  inputs=5  en=off  latency=1  precision=Full  arith_type=Unsigned  n_bits=16  bin_pt=14  quantization=Truncate  overflow=Wrap  dbl_ovrd=off  block_type=mux
  Mux6 : xbsIndex_r4/Mux  inputs=5  en=off  latency=1  precision=Full  arith_type=Unsigned  n_bits=16  bin_pt=14  quantization=Truncate  overflow=Wrap  dbl_ovrd=off  block_type=mux
  Slice_h : xbsIndex_r4/Slice  nbits=3  boolean_output=off  mode=Lower Bit Location + Width  bit1=0  base1=MSB of Input  bit0=3  base0=LSB of Input  dbl_ovrd=off  block_type=slice
  Slice_l : xbsIndex_r4/Slice  nbits=3  boolean_output=off  mode=Lower Bit Location + Width  bit1=0  base1=MSB of Input  bit0=0  base0=LSB of Input  dbl_ovrd=off  block_type=slice
  channel_select1 : InportShadow
  ca_code_out : Outport
  wires:
  [CA_code10] -> Mux2/3
  [CA_code1] -> Mux1/2
  [CA_code18] -> Mux3/3
  [CA_code11] -> Mux2/4
  Mux6/1 -> Mux4/6
  [CA_code36] -> Mux6/5
  [CA_code16] -> Mux2/9
  [CA_code25] -> Mux5/2
  [CA_code3] -> Mux1/4
  [CA_code28] -> Mux5/5
  [CA_code33] -> Mux6/2
  [CA_code13] -> Mux2/6
  Mux2/1 -> Mux4/3
  [CA_code27] -> Mux5/4
  [CA_code35] -> Mux6/4
  [CA_code5] -> Mux1/6
  [CA_code4] -> Mux1/5
  [CA_code6] -> Mux1/7
  [CA_code8] -> Mux1/9
  [CA_code20] -> Mux3/5
  Mux4/1 -> ca_code_out/1
  [CA_code9] -> Mux2/2
  Mux3/1 -> Mux4/4
  [CA_code34] -> Mux6/3
  [CA_code22] -> Mux3/7
  [CA_code30] -> Mux5/7
  [CA_code37] -> Mux6/6
  [CA_code23] -> Mux3/8
  [CA_code19] -> Mux3/4
  [CA_code2] -> Mux1/3
  [CA_code24] -> Mux3/9
  [CA_code31] -> Mux5/8
  [CA_code26] -> Mux5/3
  Mux1/1 -> Mux4/2
  [CA_code21] -> Mux3/6
  Mux5/1 -> Mux4/5
  [CA_code29] -> Mux5/6
  [CA_code14] -> Mux2/7
  [CA_code12] -> Mux2/5
  [CA_code7] -> Mux1/8
  [CA_code15] -> Mux2/8
  [CA_code32] -> Mux5/9
  [CA_code17] -> Mux3/2
  Slice_l/1 -> Mux2/1, Mux3/1, Mux5/1, Mux6/1, Mux1/1
  channel_select/1 -> Slice_l/1
  channel_select1/1 -> Slice_h/1
  Slice_h/1 -> Mux4/1

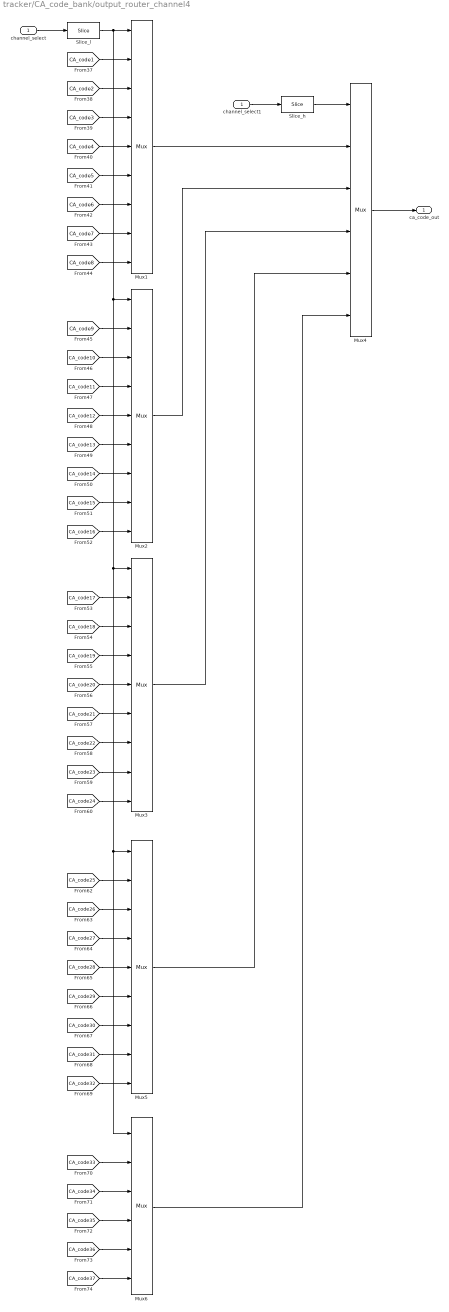
== system tracker/CA_code_bank/output_router_channel4 ==
  channel_select : Inport
  Mux{1..3,5} (4 alike) : xbsIndex_r4/Mux  inputs=8  en=off  latency=1  precision=Full  arith_type=Unsigned  n_bits=16  bin_pt=14  quantization=Truncate  overflow=Wrap  dbl_ovrd=off  block_type=mux
  Mux4 : xbsIndex_r4/Mux  inputs=5  en=off  latency=1  precision=Full  arith_type=Unsigned  n_bits=16  bin_pt=14  quantization=Truncate  overflow=Wrap  dbl_ovrd=off  block_type=mux
  Mux6 : xbsIndex_r4/Mux  inputs=5  en=off  latency=1  precision=Full  arith_type=Unsigned  n_bits=16  bin_pt=14  quantization=Truncate  overflow=Wrap  dbl_ovrd=off  block_type=mux
  Slice_h : xbsIndex_r4/Slice  nbits=3  boolean_output=off  mode=Lower Bit Location + Width  bit1=0  base1=MSB of Input  bit0=3  base0=LSB of Input  dbl_ovrd=off  block_type=slice
  Slice_l : xbsIndex_r4/Slice  nbits=3  boolean_output=off  mode=Lower Bit Location + Width  bit1=0  base1=MSB of Input  bit0=0  base0=LSB of Input  dbl_ovrd=off  block_type=slice
  channel_select1 : InportShadow
  ca_code_out : Outport
  wires:
  Slice_h/1 -> Mux4/1
  channel_select1/1 -> Slice_h/1
  channel_select/1 -> Slice_l/1
  Slice_l/1 -> Mux1/1, Mux6/1, Mux5/1, Mux3/1, Mux2/1
  [CA_code17] -> Mux3/2
  [CA_code32] -> Mux5/9
  [CA_code15] -> Mux2/8
  [CA_code7] -> Mux1/8
  [CA_code12] -> Mux2/5
  [CA_code14] -> Mux2/7
  [CA_code29] -> Mux5/6
  Mux5/1 -> Mux4/5
  [CA_code21] -> Mux3/6
  Mux1/1 -> Mux4/2
  [CA_code26] -> Mux5/3
  [CA_code31] -> Mux5/8
  [CA_code24] -> Mux3/9
  [CA_code2] -> Mux1/3
  [CA_code19] -> Mux3/4
  [CA_code23] -> Mux3/8
  [CA_code37] -> Mux6/6
  [CA_code30] -> Mux5/7
  [CA_code22] -> Mux3/7
  [CA_code34] -> Mux6/3
  Mux3/1 -> Mux4/4
  [CA_code9] -> Mux2/2
  Mux4/1 -> ca_code_out/1
  [CA_code20] -> Mux3/5
  [CA_code8] -> Mux1/9
  [CA_code6] -> Mux1/7
  [CA_code4] -> Mux1/5
  [CA_code5] -> Mux1/6
  [CA_code35] -> Mux6/4
  [CA_code27] -> Mux5/4
  Mux2/1 -> Mux4/3
  [CA_code13] -> Mux2/6
  [CA_code33] -> Mux6/2
  [CA_code28] -> Mux5/5
  [CA_code3] -> Mux1/4
  [CA_code25] -> Mux5/2
  [CA_code16] -> Mux2/9
  [CA_code36] -> Mux6/5
  Mux6/1 -> Mux4/6
  [CA_code11] -> Mux2/4
  [CA_code18] -> Mux3/3
  [CA_code1] -> Mux1/2
  [CA_code10] -> Mux2/3

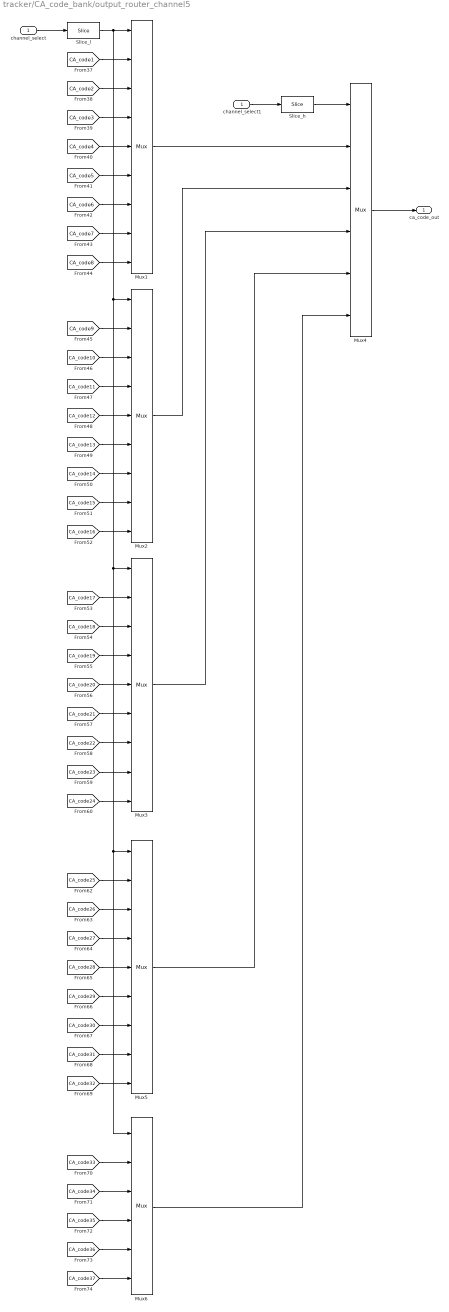
== system tracker/CA_code_bank/output_router_channel5 ==
  channel_select : Inport
  Mux{1..3,5} (4 alike) : xbsIndex_r4/Mux  inputs=8  en=off  latency=1  precision=Full  arith_type=Unsigned  n_bits=16  bin_pt=14  quantization=Truncate  overflow=Wrap  dbl_ovrd=off  block_type=mux
  Mux4 : xbsIndex_r4/Mux  inputs=5  en=off  latency=1  precision=Full  arith_type=Unsigned  n_bits=16  bin_pt=14  quantization=Truncate  overflow=Wrap  dbl_ovrd=off  block_type=mux
  Mux6 : xbsIndex_r4/Mux  inputs=5  en=off  latency=1  precision=Full  arith_type=Unsigned  n_bits=16  bin_pt=14  quantization=Truncate  overflow=Wrap  dbl_ovrd=off  block_type=mux
  Slice_h : xbsIndex_r4/Slice  nbits=3  boolean_output=off  mode=Lower Bit Location + Width  bit1=0  base1=MSB of Input  bit0=3  base0=LSB of Input  dbl_ovrd=off  block_type=slice
  Slice_l : xbsIndex_r4/Slice  nbits=3  boolean_output=off  mode=Lower Bit Location + Width  bit1=0  base1=MSB of Input  bit0=0  base0=LSB of Input  dbl_ovrd=off  block_type=slice
  channel_select1 : InportShadow
  ca_code_out : Outport
  wires:
  [CA_code10] -> Mux2/3
  [CA_code1] -> Mux1/2
  [CA_code18] -> Mux3/3
  [CA_code11] -> Mux2/4
  Mux6/1 -> Mux4/6
  [CA_code36] -> Mux6/5
  [CA_code16] -> Mux2/9
  [CA_code25] -> Mux5/2
  [CA_code3] -> Mux1/4
  [CA_code28] -> Mux5/5
  [CA_code33] -> Mux6/2
  [CA_code13] -> Mux2/6
  Mux2/1 -> Mux4/3
  [CA_code27] -> Mux5/4
  [CA_code35] -> Mux6/4
  [CA_code5] -> Mux1/6
  [CA_code4] -> Mux1/5
  [CA_code6] -> Mux1/7
  [CA_code8] -> Mux1/9
  [CA_code20] -> Mux3/5
  Mux4/1 -> ca_code_out/1
  [CA_code9] -> Mux2/2
  Mux3/1 -> Mux4/4
  [CA_code34] -> Mux6/3
  [CA_code22] -> Mux3/7
  [CA_code30] -> Mux5/7
  [CA_code37] -> Mux6/6
  [CA_code23] -> Mux3/8
  [CA_code19] -> Mux3/4
  [CA_code2] -> Mux1/3
  [CA_code24] -> Mux3/9
  [CA_code31] -> Mux5/8
  [CA_code26] -> Mux5/3
  Mux1/1 -> Mux4/2
  [CA_code21] -> Mux3/6
  Mux5/1 -> Mux4/5
  [CA_code29] -> Mux5/6
  [CA_code14] -> Mux2/7
  [CA_code12] -> Mux2/5
  [CA_code7] -> Mux1/8
  [CA_code15] -> Mux2/8
  [CA_code32] -> Mux5/9
  [CA_code17] -> Mux3/2
  Slice_l/1 -> Mux2/1, Mux3/1, Mux5/1, Mux6/1, Mux1/1
  channel_select/1 -> Slice_l/1
  channel_select1/1 -> Slice_h/1
  Slice_h/1 -> Mux4/1

== system tracker/CA_code_bank/output_router_channel6 ==
  channel_select : Inport
  Mux{1..3,5} (4 alike) : xbsIndex_r4/Mux  inputs=8  en=off  latency=1  precision=Full  arith_type=Unsigned  n_bits=16  bin_pt=14  quantization=Truncate  overflow=Wrap  dbl_ovrd=off  block_type=mux
  Mux4 : xbsIndex_r4/Mux  inputs=5  en=off  latency=1  precision=Full  arith_type=Unsigned  n_bits=16  bin_pt=14  quantization=Truncate  overflow=Wrap  dbl_ovrd=off  block_type=mux
  Mux6 : xbsIndex_r4/Mux  inputs=5  en=off  latency=1  precision=Full  arith_type=Unsigned  n_bits=16  bin_pt=14  quantization=Truncate  overflow=Wrap  dbl_ovrd=off  block_type=mux
  Slice_h : xbsIndex_r4/Slice  nbits=3  boolean_output=off  mode=Lower Bit Location + Width  bit1=0  base1=MSB of Input  bit0=3  base0=LSB of Input  dbl_ovrd=off  block_type=slice
  Slice_l : xbsIndex_r4/Slice  nbits=3  boolean_output=off  mode=Lower Bit Location + Width  bit1=0  base1=MSB of Input  bit0=0  base0=LSB of Input  dbl_ovrd=off  block_type=slice
  channel_select1 : InportShadow
  ca_code_out : Outport
  wires:
  Slice_h/1 -> Mux4/1
  channel_select1/1 -> Slice_h/1
  channel_select/1 -> Slice_l/1
  Slice_l/1 -> Mux1/1, Mux6/1, Mux5/1, Mux3/1, Mux2/1
  [CA_code17] -> Mux3/2
  [CA_code32] -> Mux5/9
  [CA_code15] -> Mux2/8
  [CA_code7] -> Mux1/8
  [CA_code12] -> Mux2/5
  [CA_code14] -> Mux2/7
  [CA_code29] -> Mux5/6
  Mux5/1 -> Mux4/5
  [CA_code21] -> Mux3/6
  Mux1/1 -> Mux4/2
  [CA_code26] -> Mux5/3
  [CA_code31] -> Mux5/8
  [CA_code24] -> Mux3/9
  [CA_code2] -> Mux1/3
  [CA_code19] -> Mux3/4
  [CA_code23] -> Mux3/8
  [CA_code37] -> Mux6/6
  [CA_code30] -> Mux5/7
  [CA_code22] -> Mux3/7
  [CA_code34] -> Mux6/3
  Mux3/1 -> Mux4/4
  [CA_code9] -> Mux2/2
  Mux4/1 -> ca_code_out/1
  [CA_code20] -> Mux3/5
  [CA_code8] -> Mux1/9
  [CA_code6] -> Mux1/7
  [CA_code4] -> Mux1/5
  [CA_code5] -> Mux1/6
  [CA_code35] -> Mux6/4
  [CA_code27] -> Mux5/4
  Mux2/1 -> Mux4/3
  [CA_code13] -> Mux2/6
  [CA_code33] -> Mux6/2
  [CA_code28] -> Mux5/5
  [CA_code3] -> Mux1/4
  [CA_code25] -> Mux5/2
  [CA_code16] -> Mux2/9
  [CA_code36] -> Mux6/5
  Mux6/1 -> Mux4/6
  [CA_code11] -> Mux2/4
  [CA_code18] -> Mux3/3
  [CA_code1] -> Mux1/2
  [CA_code10] -> Mux2/3

== system tracker/CA_code_bank/output_router_channel7 ==
  channel_select : Inport
  Mux{1..3,5} (4 alike) : xbsIndex_r4/Mux  inputs=8  en=off  latency=1  precision=Full  arith_type=Unsigned  n_bits=16  bin_pt=14  quantization=Truncate  overflow=Wrap  dbl_ovrd=off  block_type=mux
  Mux4 : xbsIndex_r4/Mux  inputs=5  en=off  latency=1  precision=Full  arith_type=Unsigned  n_bits=16  bin_pt=14  quantization=Truncate  overflow=Wrap  dbl_ovrd=off  block_type=mux
  Mux6 : xbsIndex_r4/Mux  inputs=5  en=off  latency=1  precision=Full  arith_type=Unsigned  n_bits=16  bin_pt=14  quantization=Truncate  overflow=Wrap  dbl_ovrd=off  block_type=mux
  Slice_h : xbsIndex_r4/Slice  nbits=3  boolean_output=off  mode=Lower Bit Location + Width  bit1=0  base1=MSB of Input  bit0=3  base0=LSB of Input  dbl_ovrd=off  block_type=slice
  Slice_l : xbsIndex_r4/Slice  nbits=3  boolean_output=off  mode=Lower Bit Location + Width  bit1=0  base1=MSB of Input  bit0=0  base0=LSB of Input  dbl_ovrd=off  block_type=slice
  channel_select1 : InportShadow
  ca_code_out : Outport
  wires:
  Slice_h/1 -> Mux4/1
  channel_select1/1 -> Slice_h/1
  channel_select/1 -> Slice_l/1
  Slice_l/1 -> Mux1/1, Mux6/1, Mux5/1, Mux3/1, Mux2/1
  [CA_code17] -> Mux3/2
  [CA_code32] -> Mux5/9
  [CA_code15] -> Mux2/8
  [CA_code7] -> Mux1/8
  [CA_code12] -> Mux2/5
  [CA_code14] -> Mux2/7
  [CA_code29] -> Mux5/6
  Mux5/1 -> Mux4/5
  [CA_code21] -> Mux3/6
  Mux1/1 -> Mux4/2
  [CA_code26] -> Mux5/3
  [CA_code31] -> Mux5/8
  [CA_code24] -> Mux3/9
  [CA_code2] -> Mux1/3
  [CA_code19] -> Mux3/4
  [CA_code23] -> Mux3/8
  [CA_code37] -> Mux6/6
  [CA_code30] -> Mux5/7
  [CA_code22] -> Mux3/7
  [CA_code34] -> Mux6/3
  Mux3/1 -> Mux4/4
  [CA_code9] -> Mux2/2
  Mux4/1 -> ca_code_out/1
  [CA_code20] -> Mux3/5
  [CA_code8] -> Mux1/9
  [CA_code6] -> Mux1/7
  [CA_code4] -> Mux1/5
  [CA_code5] -> Mux1/6
  [CA_code35] -> Mux6/4
  [CA_code27] -> Mux5/4
  Mux2/1 -> Mux4/3
  [CA_code13] -> Mux2/6
  [CA_code33] -> Mux6/2
  [CA_code28] -> Mux5/5
  [CA_code3] -> Mux1/4
  [CA_code25] -> Mux5/2
  [CA_code16] -> Mux2/9
  [CA_code36] -> Mux6/5
  Mux6/1 -> Mux4/6
  [CA_code11] -> Mux2/4
  [CA_code18] -> Mux3/3
  [CA_code1] -> Mux1/2
  [CA_code10] -> Mux2/3

== system tracker/CA_code_bank/output_router_channel8 ==
  channel_select : Inport
  Mux{1..3,5} (4 alike) : xbsIndex_r4/Mux  inputs=8  en=off  latency=1  precision=Full  arith_type=Unsigned  n_bits=16  bin_pt=14  quantization=Truncate  overflow=Wrap  dbl_ovrd=off  block_type=mux
  Mux4 : xbsIndex_r4/Mux  inputs=5  en=off  latency=1  precision=Full  arith_type=Unsigned  n_bits=16  bin_pt=14  quantization=Truncate  overflow=Wrap  dbl_ovrd=off  block_type=mux
  Mux6 : xbsIndex_r4/Mux  inputs=5  en=off  latency=1  precision=Full  arith_type=Unsigned  n_bits=16  bin_pt=14  quantization=Truncate  overflow=Wrap  dbl_ovrd=off  block_type=mux
  Slice_h : xbsIndex_r4/Slice  nbits=3  boolean_output=off  mode=Lower Bit Location + Width  bit1=0  base1=MSB of Input  bit0=3  base0=LSB of Input  dbl_ovrd=off  block_type=slice
  Slice_l : xbsIndex_r4/Slice  nbits=3  boolean_output=off  mode=Lower Bit Location + Width  bit1=0  base1=MSB of Input  bit0=0  base0=LSB of Input  dbl_ovrd=off  block_type=slice
  channel_select1 : InportShadow
  ca_code_out : Outport
  wires:
  [CA_code10] -> Mux2/3
  [CA_code1] -> Mux1/2
  [CA_code18] -> Mux3/3
  [CA_code11] -> Mux2/4
  Mux6/1 -> Mux4/6
  [CA_code36] -> Mux6/5
  [CA_code16] -> Mux2/9
  [CA_code25] -> Mux5/2
  [CA_code3] -> Mux1/4
  [CA_code28] -> Mux5/5
  [CA_code33] -> Mux6/2
  [CA_code13] -> Mux2/6
  Mux2/1 -> Mux4/3
  [CA_code27] -> Mux5/4
  [CA_code35] -> Mux6/4
  [CA_code5] -> Mux1/6
  [CA_code4] -> Mux1/5
  [CA_code6] -> Mux1/7
  [CA_code8] -> Mux1/9
  [CA_code20] -> Mux3/5
  Mux4/1 -> ca_code_out/1
  [CA_code9] -> Mux2/2
  Mux3/1 -> Mux4/4
  [CA_code34] -> Mux6/3
  [CA_code22] -> Mux3/7
  [CA_code30] -> Mux5/7
  [CA_code37] -> Mux6/6
  [CA_code23] -> Mux3/8
  [CA_code19] -> Mux3/4
  [CA_code2] -> Mux1/3
  [CA_code24] -> Mux3/9
  [CA_code31] -> Mux5/8
  [CA_code26] -> Mux5/3
  Mux1/1 -> Mux4/2
  [CA_code21] -> Mux3/6
  Mux5/1 -> Mux4/5
  [CA_code29] -> Mux5/6
  [CA_code14] -> Mux2/7
  [CA_code12] -> Mux2/5
  [CA_code7] -> Mux1/8
  [CA_code15] -> Mux2/8
  [CA_code32] -> Mux5/9
  [CA_code17] -> Mux3/2
  Slice_l/1 -> Mux2/1, Mux3/1, Mux5/1, Mux6/1, Mux1/1
  channel_select/1 -> Slice_l/1
  channel_select1/1 -> Slice_h/1
  Slice_h/1 -> Mux4/1

== system tracker/CA_code_bank/output_router_channel9 ==
  channel_select : Inport
  Mux{1..3,5} (4 alike) : xbsIndex_r4/Mux  inputs=8  en=off  latency=1  precision=Full  arith_type=Unsigned  n_bits=16  bin_pt=14  quantization=Truncate  overflow=Wrap  dbl_ovrd=off  block_type=mux
  Mux4 : xbsIndex_r4/Mux  inputs=5  en=off  latency=1  precision=Full  arith_type=Unsigned  n_bits=16  bin_pt=14  quantization=Truncate  overflow=Wrap  dbl_ovrd=off  block_type=mux
  Mux6 : xbsIndex_r4/Mux  inputs=5  en=off  latency=1  precision=Full  arith_type=Unsigned  n_bits=16  bin_pt=14  quantization=Truncate  overflow=Wrap  dbl_ovrd=off  block_type=mux
  Slice_h : xbsIndex_r4/Slice  nbits=3  boolean_output=off  mode=Lower Bit Location + Width  bit1=0  base1=MSB of Input  bit0=3  base0=LSB of Input  dbl_ovrd=off  block_type=slice
  Slice_l : xbsIndex_r4/Slice  nbits=3  boolean_output=off  mode=Lower Bit Location + Width  bit1=0  base1=MSB of Input  bit0=0  base0=LSB of Input  dbl_ovrd=off  block_type=slice
  channel_select1 : InportShadow
  ca_code_out : Outport
  wires:
  Slice_h/1 -> Mux4/1
  channel_select1/1 -> Slice_h/1
  channel_select/1 -> Slice_l/1
  Slice_l/1 -> Mux1/1, Mux6/1, Mux5/1, Mux3/1, Mux2/1
  [CA_code17] -> Mux3/2
  [CA_code32] -> Mux5/9
  [CA_code15] -> Mux2/8
  [CA_code7] -> Mux1/8
  [CA_code12] -> Mux2/5
  [CA_code14] -> Mux2/7
  [CA_code29] -> Mux5/6
  Mux5/1 -> Mux4/5
  [CA_code21] -> Mux3/6
  Mux1/1 -> Mux4/2
  [CA_code26] -> Mux5/3
  [CA_code31] -> Mux5/8
  [CA_code24] -> Mux3/9
  [CA_code2] -> Mux1/3
  [CA_code19] -> Mux3/4
  [CA_code23] -> Mux3/8
  [CA_code37] -> Mux6/6
  [CA_code30] -> Mux5/7
  [CA_code22] -> Mux3/7
  [CA_code34] -> Mux6/3
  Mux3/1 -> Mux4/4
  [CA_code9] -> Mux2/2
  Mux4/1 -> ca_code_out/1
  [CA_code20] -> Mux3/5
  [CA_code8] -> Mux1/9
  [CA_code6] -> Mux1/7
  [CA_code4] -> Mux1/5
  [CA_code5] -> Mux1/6
  [CA_code35] -> Mux6/4
  [CA_code27] -> Mux5/4
  Mux2/1 -> Mux4/3
  [CA_code13] -> Mux2/6
  [CA_code33] -> Mux6/2
  [CA_code28] -> Mux5/5
  [CA_code3] -> Mux1/4
  [CA_code25] -> Mux5/2
  [CA_code16] -> Mux2/9
  [CA_code36] -> Mux6/5
  Mux6/1 -> Mux4/6
  [CA_code11] -> Mux2/4
  [CA_code18] -> Mux3/3
  [CA_code1] -> Mux1/2
  [CA_code10] -> Mux2/3

== system tracker/code_carrier_tracking_loop1/carrier_loop_discriminator ==
  Ips : Inport
  Qps : Inport  Port=2
  loop_filter : Subsystem
  pll_discriminators : Subsystem
  Out1 : Outport
  wires:
  Ips/1 -> pll_discriminators/1(I)
  Qps/1 -> pll_discriminators/2(Q)
  pll_discriminators/1(phi) -> loop_filter/1(phi)

== system tracker/code_carrier_tracking_loop1/code_loop_discriminator ==
  Ies : Inport
  Ils : Inport  Port=2
  Qes : Inport  Port=3
  Qls : Inport  Port=4
  DLL_Discriminators : Subsystem
  Out1 : Outport
  wires:
  Ies/1 -> DLL_Discriminators/1(Ies)
  DLL_Discriminators/1(sdfa) -> Out1/1
  Qes/1 -> DLL_Discriminators/2(Qes)
  Ils/1 -> DLL_Discriminators/3(Ils)
  Qls/1 -> DLL_Discriminators/4(Qls)

== system tracker/code_carrier_tracking_loop1/integration_and_dump_ie ==
  data_in : Inport
  add_sub : Inport  Port=2
  reset : Inport  Port=3
  AddSub : xbsIndex_r4/AddSub  mode=Addition or Subtraction  use_carryin=off  use_carryout=off  en=off  latency=0  precision=User Defined  arith_type="Signed  (2's comp)"  n_bits=integration_acc_width  bin_pt=integration_acc_point  quantization="Round  (unbiased: +/- Inf)"  overflow=Saturate  use_behavioral_HDL=off  hw_selection=Fabric  pipelined=off  dbl_ovrd=off  block_type=addsub
  Register30 : xbsIndex_r4/Register  init=0  rst=on  en=off  dbl_ovrd=off  block_type=register
  data_out : Outport
  wires:
  reset/1 -> Register30/2
  AddSub/1 -> Register30/1
  data_in/1 -> AddSub/2
  add_sub/1 -> AddSub/3
  Register30/1 -> data_out/1, AddSub/1

== system tracker/code_carrier_tracking_loop1/integration_and_dump_il ==
  data_in : Inport
  add_sub : Inport  Port=2
  reset : Inport  Port=3
  AddSub : xbsIndex_r4/AddSub  mode=Addition or Subtraction  use_carryin=off  use_carryout=off  en=off  latency=0  precision=User Defined  arith_type="Signed  (2's comp)"  n_bits=integration_acc_width  bin_pt=integration_acc_point  quantization="Round  (unbiased: +/- Inf)"  overflow=Saturate  use_behavioral_HDL=off  hw_selection=Fabric  pipelined=off  dbl_ovrd=off  block_type=addsub
  Register30 : xbsIndex_r4/Register  init=0  rst=on  en=off  dbl_ovrd=off  block_type=register
  data_out : Outport
  wires:
  reset/1 -> Register30/2
  AddSub/1 -> Register30/1
  data_in/1 -> AddSub/2
  add_sub/1 -> AddSub/3
  Register30/1 -> data_out/1, AddSub/1

== system tracker/code_carrier_tracking_loop1/integration_and_dump_ip ==
  data_in : Inport
  add_sub : Inport  Port=2
  reset : Inport  Port=3
  AddSub : xbsIndex_r4/AddSub  mode=Addition or Subtraction  use_carryin=off  use_carryout=off  en=off  latency=0  precision=User Defined  arith_type="Signed  (2's comp)"  n_bits=integration_acc_width  bin_pt=integration_acc_point  quantization="Round  (unbiased: +/- Inf)"  overflow=Saturate  use_behavioral_HDL=off  hw_selection=Fabric  pipelined=off  dbl_ovrd=off  block_type=addsub
  Register30 : xbsIndex_r4/Register  init=0  rst=on  en=off  dbl_ovrd=off  block_type=register
  data_out : Outport
  wires:
  Register30/1 -> AddSub/1, data_out/1
  add_sub/1 -> AddSub/3
  data_in/1 -> AddSub/2
  AddSub/1 -> Register30/1
  reset/1 -> Register30/2

== system tracker/code_carrier_tracking_loop1/integration_and_dump_qe ==
  data_in : Inport
  add_sub : Inport  Port=2
  reset : Inport  Port=3
  AddSub : xbsIndex_r4/AddSub  mode=Addition or Subtraction  use_carryin=off  use_carryout=off  en=off  latency=0  precision=User Defined  arith_type="Signed  (2's comp)"  n_bits=integration_acc_width  bin_pt=integration_acc_point  quantization="Round  (unbiased: +/- Inf)"  overflow=Saturate  use_behavioral_HDL=off  hw_selection=Fabric  pipelined=off  dbl_ovrd=off  block_type=addsub
  Register30 : xbsIndex_r4/Register  init=0  rst=on  en=off  dbl_ovrd=off  block_type=register
  data_out : Outport
  wires:
  Register30/1 -> AddSub/1, data_out/1
  add_sub/1 -> AddSub/3
  data_in/1 -> AddSub/2
  AddSub/1 -> Register30/1
  reset/1 -> Register30/2

== system tracker/code_carrier_tracking_loop1/integration_and_dump_ql ==
  data_in : Inport
  add_sub : Inport  Port=2
  reset : Inport  Port=3
  AddSub : xbsIndex_r4/AddSub  mode=Addition or Subtraction  use_carryin=off  use_carryout=off  en=off  latency=0  precision=User Defined  arith_type="Signed  (2's comp)"  n_bits=integration_acc_width  bin_pt=integration_acc_point  quantization="Round  (unbiased: +/- Inf)"  overflow=Saturate  use_behavioral_HDL=off  hw_selection=Fabric  pipelined=off  dbl_ovrd=off  block_type=addsub
  Register30 : xbsIndex_r4/Register  init=0  rst=on  en=off  dbl_ovrd=off  block_type=register
  data_out : Outport
  wires:
  Register30/1 -> AddSub/1, data_out/1
  add_sub/1 -> AddSub/3
  data_in/1 -> AddSub/2
  AddSub/1 -> Register30/1
  reset/1 -> Register30/2

== system tracker/code_carrier_tracking_loop1/integration_and_dump_qp ==
  data_in : Inport
  add_sub : Inport  Port=2
  reset : Inport  Port=3
  AddSub : xbsIndex_r4/AddSub  mode=Addition or Subtraction  use_carryin=off  use_carryout=off  en=off  latency=0  precision=User Defined  arith_type="Signed  (2's comp)"  n_bits=integration_acc_width  bin_pt=integration_acc_point  quantization="Round  (unbiased: +/- Inf)"  overflow=Saturate  use_behavioral_HDL=off  hw_selection=Fabric  pipelined=off  dbl_ovrd=off  block_type=addsub
  Register30 : xbsIndex_r4/Register  init=0  rst=on  en=off  dbl_ovrd=off  block_type=register
  data_out : Outport
  wires:
  reset/1 -> Register30/2
  AddSub/1 -> Register30/1
  data_in/1 -> AddSub/2
  add_sub/1 -> AddSub/3
  Register30/1 -> data_out/1, AddSub/1
